simulink model "GFLI_L"  (R2024b)
settings: Solver=ode4  StartTime=0.0  StopTime=Tsim  FixedStep=Tsam  RelTol=1e-3
values from neighbouring files (symbols this model uses):
  Tsam = 5e-5    (= 5e-05)    [generate_ibr_impedance_datasets_param_casegrid_memorysafe.m]
  w_meas = 2*pi*fHz_meas(:)    [generate_ibr_impedance_datasets_param_casegrid_memorysafe.m]
undefined symbols (not defined in the file or in its folder): DiscIntNeverNeededParam, I2d, I2q, Kii, Kipll, Kpi, Kppll, Lf1, Rf1, Td, Vdc, Vg, w, w1
libraries: slctrl_fre x12, spsControlledVoltageSourceLib x6, spsabctodq0Lib x5, slctrl_signal x4, spsACVoltageSourceLib x3, spsSeriesRLCBranchLib x3, spsdq0toabcLib x2, spsThreePhaseVIMeasurementLib x2, spsPLL3phLib x1, spsGroundLib x1, sps_lib x1
(part 2 of 2)

== system GFLI_L/Data Logging for 'frestimate'1/Generate Info Signal/Superposition ==
  start/stop : Inport
  Info Bus : BusCreator  Inputs=1
  Info Snapshot : slctrl_fre/Frequency Response Estimator/Frequency Response Estimator/Variant Subsystem/PRBSNoEst/Info Snapshot  SystemSampleTime=-1  VariantActivationTime=update diagram  AllowFlexibleInterface=on  Latency=0  AutoFrameSizeCalculation=off
  conversion factor : Gain  Gain=ConvFactor
  frequencies : Constant  Value=FrequenciesSI  SampleTime=Ts
  Info : Outport
  wires:
  conversion factor/1 -> Info Snapshot/1
  Info Bus/1 -> Info/1  "Info"
  start/stop/1 -> Info Snapshot/Enable
  frequencies/1 -> conversion factor/1
  Info Snapshot/1 -> Info Bus/1  "frequencies"

== system GFLI_L/Data Logging for 'frestimate'1/Generate Ready Signal/PRBS ==
  Freq Index : Inport
  Perturbation : Inport  Port=2
  Constant : Constant  Value=0  SampleTime=Ts
  Relational Operator : RelationalOperator  Operator=~=  OutDataTypeStr=boolean  RndMeth=Simplest  InputSameDT=off
  Terminator : Terminator
  Ready : Outport
  wires:
  Relational Operator/1 -> Ready/1  "Ready"
  Constant/1 -> Relational Operator/2
  Perturbation/1 -> Relational Operator/1  "Perturbation"
  Freq Index/1 -> Terminator/1

== system GFLI_L/Data Logging for 'frestimate'1/Generate Ready Signal/Sinestream ==
  Freq Index : Inport
  Perturbation : Inport  Port=2
  ExtractReadySignal : Subsystem  mask(Extract Ready Signal){Ts=Ts, Frequencies=FrequenciesSS, NumOfSetPeriod=NumOfSetPeriod, NumOfEstPeriod=NumOfEstPeriod}
      mask prompts: Ts "Sample Time (Ts)"; Frequencies "Frequencies Vector"; NumOfSetPeriod "Number of Settling Periods"; NumOfEstPeriod "Number of Estimation Periods"
      mask help: Extract ready signal for the Sinestream Signal Generator block for offline frequency response estimation.
      mask init:
      | nw = length(Frequencies);
  Terminator : Terminator
  Ready : Outport
  wires:
  Freq Index/1 -> ExtractReadySignal/1(Frequency Index)
  Perturbation/1 -> Terminator/1
  ExtractReadySignal/1(Ready Signal) -> Ready/1  "Ready"

== system GFLI_L/Data Logging for 'frestimate'1/Generate Ready Signal/Superposition ==
  Freq Index : Inport
  Perturbation : Inport  Port=2
  Constant : Constant  Value=0  SampleTime=Ts
  Relational Operator : RelationalOperator  Operator=~=  OutDataTypeStr=boolean  RndMeth=Simplest  InputSameDT=off
  Terminator : Terminator
  Ready : Outport
  wires:
  Freq Index/1 -> Terminator/1
  Perturbation/1 -> Relational Operator/1  "Perturbation"
  Constant/1 -> Relational Operator/2
  Relational Operator/1 -> Ready/1  "Ready"

== system GFLI_L/Data Logging for 'frestimate'1/Subtract Nominal Values/Enabled Subsystem ==
  u : Inport
  y : Inport  Port=2
  start/stop : Inport  Port=3
  Enable : EnablePort
  ExtractNominalValues : Subsystem  mask(Remove Nominal Signal){Ts=Ts}
      mask prompts: Ts "Samplt Time (sec)"
      mask help: Remove nominal baseline signal from logged data.
  Sum : Sum  Inputs=|+-
  Sum1 : Sum  Inputs=-+|
  PlantInput : Outport
  PlantOutput : Outport  Port=2
  wires:
  Sum1/1 -> PlantOutput/1
  y/1 -> ExtractNominalValues/2(y), Sum1/2
  ExtractNominalValues/2(yNominal) -> Sum1/1
  u/1 -> ExtractNominalValues/1(u), Sum/1
  ExtractNominalValues/1(uNominal) -> Sum/2
  Sum/1 -> PlantInput/1
  start/stop/1 -> ExtractNominalValues/3(start/stop)

== system GFLI_L/Data Logging for 'frestimate'2/Generate Info Signal/PRBS ==
  start/stop : Inport
  Info Bus : BusCreator  Inputs=1
  Info Snapshot : slctrl_fre/Frequency Response Estimator/Frequency Response Estimator/Variant Subsystem/PRBSNoEst/Info Snapshot  SystemSampleTime=-1  VariantActivationTime=update diagram  AllowFlexibleInterface=on  Latency=0  AutoFrameSizeCalculation=off
  PRBSNumPeriods : Constant  Value=PRBSNumOfPeriod  SampleTime=Ts
  Info : Outport
  wires:
  PRBSNumPeriods/1 -> Info Snapshot/1
  Info Bus/1 -> Info/1  "Info"
  Info Snapshot/1 -> Info Bus/1  "PRBSNumPeriods"
  start/stop/1 -> Info Snapshot/Enable

== system GFLI_L/Data Logging for 'frestimate'2/Generate Info Signal/Sinestream ==
  start/stop : Inport
  Info Bus : BusCreator  Inputs=1
  Info Snapshot : slctrl_fre/Frequency Response Estimator/Frequency Response Estimator/Variant Subsystem/PRBSNoEst/Info Snapshot  SystemSampleTime=-1  VariantActivationTime=update diagram  AllowFlexibleInterface=on  Latency=0  AutoFrameSizeCalculation=off
  conversion factor : Gain  Gain=ConvFactor
  frequencies : Constant  Value=FrequenciesSS  SampleTime=Ts
  Info : Outport
  wires:
  conversion factor/1 -> Info Snapshot/1
  Info Snapshot/1 -> Info Bus/1  "frequencies"
  frequencies/1 -> conversion factor/1
  start/stop/1 -> Info Snapshot/Enable
  Info Bus/1 -> Info/1  "Info"

== system GFLI_L/Data Logging for 'frestimate'2/Generate Info Signal/Superposition ==
  start/stop : Inport
  Info Bus : BusCreator  Inputs=1
  Info Snapshot : slctrl_fre/Frequency Response Estimator/Frequency Response Estimator/Variant Subsystem/PRBSNoEst/Info Snapshot  SystemSampleTime=-1  VariantActivationTime=update diagram  AllowFlexibleInterface=on  Latency=0  AutoFrameSizeCalculation=off
  conversion factor : Gain  Gain=ConvFactor
  frequencies : Constant  Value=FrequenciesSI  SampleTime=Ts
  Info : Outport
  wires:
  conversion factor/1 -> Info Snapshot/1
  Info Bus/1 -> Info/1  "Info"
  start/stop/1 -> Info Snapshot/Enable
  frequencies/1 -> conversion factor/1
  Info Snapshot/1 -> Info Bus/1  "frequencies"

== system GFLI_L/Data Logging for 'frestimate'2/Generate Ready Signal/PRBS ==
  Freq Index : Inport
  Perturbation : Inport  Port=2
  Constant : Constant  Value=0  SampleTime=Ts
  Relational Operator : RelationalOperator  Operator=~=  OutDataTypeStr=boolean  RndMeth=Simplest  InputSameDT=off
  Terminator : Terminator
  Ready : Outport
  wires:
  Relational Operator/1 -> Ready/1  "Ready"
  Constant/1 -> Relational Operator/2
  Perturbation/1 -> Relational Operator/1  "Perturbation"
  Freq Index/1 -> Terminator/1

== system GFLI_L/Data Logging for 'frestimate'2/Generate Ready Signal/Sinestream ==
  Freq Index : Inport
  Perturbation : Inport  Port=2
  ExtractReadySignal : Subsystem  mask(Extract Ready Signal){Ts=Ts, Frequencies=FrequenciesSS, NumOfSetPeriod=NumOfSetPeriod, NumOfEstPeriod=NumOfEstPeriod}
      mask prompts: Ts "Sample Time (Ts)"; Frequencies "Frequencies Vector"; NumOfSetPeriod "Number of Settling Periods"; NumOfEstPeriod "Number of Estimation Periods"
      mask help: Extract ready signal for the Sinestream Signal Generator block for offline frequency response estimation.
      mask init:
      | nw = length(Frequencies);
  Terminator : Terminator
  Ready : Outport
  wires:
  Freq Index/1 -> ExtractReadySignal/1(Frequency Index)
  Perturbation/1 -> Terminator/1
  ExtractReadySignal/1(Ready Signal) -> Ready/1  "Ready"

== system GFLI_L/Data Logging for 'frestimate'2/Generate Ready Signal/Superposition ==
  Freq Index : Inport
  Perturbation : Inport  Port=2
  Constant : Constant  Value=0  SampleTime=Ts
  Relational Operator : RelationalOperator  Operator=~=  OutDataTypeStr=boolean  RndMeth=Simplest  InputSameDT=off
  Terminator : Terminator
  Ready : Outport
  wires:
  Freq Index/1 -> Terminator/1
  Perturbation/1 -> Relational Operator/1  "Perturbation"
  Constant/1 -> Relational Operator/2
  Relational Operator/1 -> Ready/1  "Ready"

== system GFLI_L/Data Logging for 'frestimate'2/Subtract Nominal Values/Enabled Subsystem ==
  u : Inport
  y : Inport  Port=2
  start/stop : Inport  Port=3
  Enable : EnablePort
  ExtractNominalValues : Subsystem  mask(Remove Nominal Signal){Ts=Ts}
      mask prompts: Ts "Samplt Time (sec)"
      mask help: Remove nominal baseline signal from logged data.
  Sum : Sum  Inputs=|+-
  Sum1 : Sum  Inputs=-+|
  PlantInput : Outport
  PlantOutput : Outport  Port=2
  wires:
  Sum1/1 -> PlantOutput/1
  y/1 -> ExtractNominalValues/2(y), Sum1/2
  ExtractNominalValues/2(yNominal) -> Sum1/1
  u/1 -> ExtractNominalValues/1(u), Sum/1
  ExtractNominalValues/1(uNominal) -> Sum/2
  Sum/1 -> PlantInput/1
  start/stop/1 -> ExtractNominalValues/3(start/stop)

== system GFLI_L/Data Logging for 'frestimate'3/Generate Info Signal/PRBS ==
  start/stop : Inport
  Info Bus : BusCreator  Inputs=1
  Info Snapshot : slctrl_fre/Frequency Response Estimator/Frequency Response Estimator/Variant Subsystem/PRBSNoEst/Info Snapshot  SystemSampleTime=-1  VariantActivationTime=update diagram  AllowFlexibleInterface=on  Latency=0  AutoFrameSizeCalculation=off
  PRBSNumPeriods : Constant  Value=PRBSNumOfPeriod  SampleTime=Ts
  Info : Outport
  wires:
  start/stop/1 -> Info Snapshot/Enable
  Info Snapshot/1 -> Info Bus/1  "PRBSNumPeriods"
  Info Bus/1 -> Info/1  "Info"
  PRBSNumPeriods/1 -> Info Snapshot/1

== system GFLI_L/Data Logging for 'frestimate'3/Generate Info Signal/Sinestream ==
  start/stop : Inport
  Info Bus : BusCreator  Inputs=1
  Info Snapshot : slctrl_fre/Frequency Response Estimator/Frequency Response Estimator/Variant Subsystem/PRBSNoEst/Info Snapshot  SystemSampleTime=-1  VariantActivationTime=update diagram  AllowFlexibleInterface=on  Latency=0  AutoFrameSizeCalculation=off
  conversion factor : Gain  Gain=ConvFactor
  frequencies : Constant  Value=FrequenciesSS  SampleTime=Ts
  Info : Outport
  wires:
  Info Bus/1 -> Info/1  "Info"
  start/stop/1 -> Info Snapshot/Enable
  frequencies/1 -> conversion factor/1
  Info Snapshot/1 -> Info Bus/1  "frequencies"
  conversion factor/1 -> Info Snapshot/1

== system GFLI_L/Data Logging for 'frestimate'3/Generate Info Signal/Superposition ==
  start/stop : Inport
  Info Bus : BusCreator  Inputs=1
  Info Snapshot : slctrl_fre/Frequency Response Estimator/Frequency Response Estimator/Variant Subsystem/PRBSNoEst/Info Snapshot  SystemSampleTime=-1  VariantActivationTime=update diagram  AllowFlexibleInterface=on  Latency=0  AutoFrameSizeCalculation=off
  conversion factor : Gain  Gain=ConvFactor
  frequencies : Constant  Value=FrequenciesSI  SampleTime=Ts
  Info : Outport
  wires:
  Info Snapshot/1 -> Info Bus/1  "frequencies"
  frequencies/1 -> conversion factor/1
  start/stop/1 -> Info Snapshot/Enable
  Info Bus/1 -> Info/1  "Info"
  conversion factor/1 -> Info Snapshot/1

== system GFLI_L/Data Logging for 'frestimate'3/Generate Ready Signal/PRBS ==
  Freq Index : Inport
  Perturbation : Inport  Port=2
  Constant : Constant  Value=0  SampleTime=Ts
  Relational Operator : RelationalOperator  Operator=~=  OutDataTypeStr=boolean  RndMeth=Simplest  InputSameDT=off
  Terminator : Terminator
  Ready : Outport
  wires:
  Freq Index/1 -> Terminator/1
  Perturbation/1 -> Relational Operator/1  "Perturbation"
  Constant/1 -> Relational Operator/2
  Relational Operator/1 -> Ready/1  "Ready"

== system GFLI_L/Data Logging for 'frestimate'3/Generate Ready Signal/Sinestream ==
  Freq Index : Inport
  Perturbation : Inport  Port=2
  ExtractReadySignal : Subsystem  mask(Extract Ready Signal){Ts=Ts, Frequencies=FrequenciesSS, NumOfSetPeriod=NumOfSetPeriod, NumOfEstPeriod=NumOfEstPeriod}
      mask prompts: Ts "Sample Time (Ts)"; Frequencies "Frequencies Vector"; NumOfSetPeriod "Number of Settling Periods"; NumOfEstPeriod "Number of Estimation Periods"
      mask help: Extract ready signal for the Sinestream Signal Generator block for offline frequency response estimation.
      mask init:
      | nw = length(Frequencies);
  Terminator : Terminator
  Ready : Outport
  wires:
  ExtractReadySignal/1(Ready Signal) -> Ready/1  "Ready"
  Perturbation/1 -> Terminator/1
  Freq Index/1 -> ExtractReadySignal/1(Frequency Index)

== system GFLI_L/Data Logging for 'frestimate'3/Generate Ready Signal/Superposition ==
  Freq Index : Inport
  Perturbation : Inport  Port=2
  Constant : Constant  Value=0  SampleTime=Ts
  Relational Operator : RelationalOperator  Operator=~=  OutDataTypeStr=boolean  RndMeth=Simplest  InputSameDT=off
  Terminator : Terminator
  Ready : Outport
  wires:
  Relational Operator/1 -> Ready/1  "Ready"
  Constant/1 -> Relational Operator/2
  Perturbation/1 -> Relational Operator/1  "Perturbation"
  Freq Index/1 -> Terminator/1

== system GFLI_L/Data Logging for 'frestimate'3/Subtract Nominal Values/Enabled Subsystem ==
  u : Inport
  y : Inport  Port=2
  start/stop : Inport  Port=3
  Enable : EnablePort
  ExtractNominalValues : Subsystem  mask(Remove Nominal Signal){Ts=Ts}
      mask prompts: Ts "Samplt Time (sec)"
      mask help: Remove nominal baseline signal from logged data.
  Sum : Sum  Inputs=|+-
  Sum1 : Sum  Inputs=-+|
  PlantInput : Outport
  PlantOutput : Outport  Port=2
  wires:
  start/stop/1 -> ExtractNominalValues/3(start/stop)
  Sum/1 -> PlantInput/1
  ExtractNominalValues/1(uNominal) -> Sum/2
  u/1 -> Sum/1, ExtractNominalValues/1(u)
  ExtractNominalValues/2(yNominal) -> Sum1/1
  y/1 -> Sum1/2, ExtractNominalValues/2(y)
  Sum1/1 -> PlantOutput/1

== system GFLI_L/Data Logging for 'frestimate'/Generate Ready Signal/Sinestream/ExtractReadySignal ==
  Frequency Index : Inport
  Est Period : Constant  Value=NumOfEstPeriod  OutDataTypeStr=double
  MATLAB Function : MATLAB Function  TreatAsAtomicUnit=on
  Numest Scalar Expansion : Gain  Gain=ones(nw,1)
  Numset Scalar Expansion : Gain  Gain=ones(nw,1)
  Set Period : Constant  Value=NumOfSetPeriod  OutDataTypeStr=double
  Triggered Subsystem : Subsystem  TreatAsAtomicUnit=on
  sample time : Constant  Value=Ts  OutDataTypeStr=double
  w constant : Constant  Value=FrequenciesSS  OutDataTypeStr=double
  Ready Signal : Outport
  wires:
  sample time/1 -> MATLAB Function/2(Ts)
  Numest Scalar Expansion/1 -> MATLAB Function/3(NumOfEstPeriod)
  w constant/1 -> MATLAB Function/1(Frequencies)
  MATLAB Function/1(Tf) -> Triggered Subsystem/2(Tf)
  Est Period/1 -> Numest Scalar Expansion/1
  Numset Scalar Expansion/1 -> MATLAB Function/4(NumOfSetPeriod)
  Frequency Index/1 -> Triggered Subsystem/1(index), Triggered Subsystem/Enable
  Triggered Subsystem/1(Ready) -> Ready Signal/1
  Set Period/1 -> Numset Scalar Expansion/1
  MATLAB Function/2(tstart) -> Triggered Subsystem/3(tstart)
  MATLAB Function/3(tsettling) -> Triggered Subsystem/4(tsettling)

== system GFLI_L/Data Logging for 'frestimate'/Subtract Nominal Values/Enabled Subsystem/ExtractNominalValues ==
  u : Inport
  y : Inport  Port=2
  start/stop : Inport  Port=3
  DisplayU0 : Display
  DisplayY0 : Display
  Enabled Delay U : Delay  DelayLength=1  InitialConditionSource=Input port  ExternalReset=Rising  SampleTime=Ts
      settings: InputPortMap=u0,r5,p4
  Enabled Delay Y : Delay  DelayLength=1  InitialConditionSource=Input port  ExternalReset=Rising  SampleTime=Ts
      settings: InputPortMap=u0,r5,p4
  uNominal : Outport  OutDataTypeStr=double  VectorParamsAs1DForOutWhenUnconnected=off
  yNominal : Outport  Port=2  OutDataTypeStr=double  VectorParamsAs1DForOutWhenUnconnected=off
  wires:
  Enabled Delay U/1 -> uNominal/1, DisplayU0/1, Enabled Delay U/1  "u"
  Enabled Delay Y/1 -> yNominal/1, Enabled Delay Y/1, DisplayY0/1  "y"
  start/stop/1 -> Enabled Delay Y/2, Enabled Delay U/2
  u/1 -> Enabled Delay U/3
  y/1 -> Enabled Delay Y/3

== system GFLI_L/Data Logging for 'frestimate'1/Generate Ready Signal/Sinestream/ExtractReadySignal ==
  Frequency Index : Inport
  Est Period : Constant  Value=NumOfEstPeriod  OutDataTypeStr=double
  MATLAB Function : MATLAB Function  TreatAsAtomicUnit=on
  Numest Scalar Expansion : Gain  Gain=ones(nw,1)
  Numset Scalar Expansion : Gain  Gain=ones(nw,1)
  Set Period : Constant  Value=NumOfSetPeriod  OutDataTypeStr=double
  Triggered Subsystem : Subsystem  TreatAsAtomicUnit=on
  sample time : Constant  Value=Ts  OutDataTypeStr=double
  w constant : Constant  Value=FrequenciesSS  OutDataTypeStr=double
  Ready Signal : Outport
  wires:
  MATLAB Function/3(tsettling) -> Triggered Subsystem/4(tsettling)
  MATLAB Function/2(tstart) -> Triggered Subsystem/3(tstart)
  Set Period/1 -> Numset Scalar Expansion/1
  Triggered Subsystem/1(Ready) -> Ready Signal/1
  Frequency Index/1 -> Triggered Subsystem/Enable, Triggered Subsystem/1(index)
  Numset Scalar Expansion/1 -> MATLAB Function/4(NumOfSetPeriod)
  Est Period/1 -> Numest Scalar Expansion/1
  MATLAB Function/1(Tf) -> Triggered Subsystem/2(Tf)
  w constant/1 -> MATLAB Function/1(Frequencies)
  Numest Scalar Expansion/1 -> MATLAB Function/3(NumOfEstPeriod)
  sample time/1 -> MATLAB Function/2(Ts)

== system GFLI_L/Data Logging for 'frestimate'1/Subtract Nominal Values/Enabled Subsystem/ExtractNominalValues ==
  u : Inport
  y : Inport  Port=2
  start/stop : Inport  Port=3
  DisplayU0 : Display
  DisplayY0 : Display
  Enabled Delay U : Delay  DelayLength=1  InitialConditionSource=Input port  ExternalReset=Rising  SampleTime=Ts
      settings: InputPortMap=u0,r5,p4
  Enabled Delay Y : Delay  DelayLength=1  InitialConditionSource=Input port  ExternalReset=Rising  SampleTime=Ts
      settings: InputPortMap=u0,r5,p4
  uNominal : Outport  OutDataTypeStr=double  VectorParamsAs1DForOutWhenUnconnected=off
  yNominal : Outport  Port=2  OutDataTypeStr=double  VectorParamsAs1DForOutWhenUnconnected=off
  wires:
  y/1 -> Enabled Delay Y/3
  u/1 -> Enabled Delay U/3
  start/stop/1 -> Enabled Delay U/2, Enabled Delay Y/2
  Enabled Delay Y/1 -> DisplayY0/1, Enabled Delay Y/1, yNominal/1  "y"
  Enabled Delay U/1 -> Enabled Delay U/1, DisplayU0/1, uNominal/1  "u"

== system GFLI_L/Data Logging for 'frestimate'2/Generate Ready Signal/Sinestream/ExtractReadySignal ==
  Frequency Index : Inport
  Est Period : Constant  Value=NumOfEstPeriod  OutDataTypeStr=double
  MATLAB Function : MATLAB Function  TreatAsAtomicUnit=on
  Numest Scalar Expansion : Gain  Gain=ones(nw,1)
  Numset Scalar Expansion : Gain  Gain=ones(nw,1)
  Set Period : Constant  Value=NumOfSetPeriod  OutDataTypeStr=double
  Triggered Subsystem : Subsystem  TreatAsAtomicUnit=on
  sample time : Constant  Value=Ts  OutDataTypeStr=double
  w constant : Constant  Value=FrequenciesSS  OutDataTypeStr=double
  Ready Signal : Outport
  wires:
  MATLAB Function/3(tsettling) -> Triggered Subsystem/4(tsettling)
  MATLAB Function/2(tstart) -> Triggered Subsystem/3(tstart)
  Set Period/1 -> Numset Scalar Expansion/1
  Triggered Subsystem/1(Ready) -> Ready Signal/1
  Frequency Index/1 -> Triggered Subsystem/Enable, Triggered Subsystem/1(index)
  Numset Scalar Expansion/1 -> MATLAB Function/4(NumOfSetPeriod)
  Est Period/1 -> Numest Scalar Expansion/1
  MATLAB Function/1(Tf) -> Triggered Subsystem/2(Tf)
  w constant/1 -> MATLAB Function/1(Frequencies)
  Numest Scalar Expansion/1 -> MATLAB Function/3(NumOfEstPeriod)
  sample time/1 -> MATLAB Function/2(Ts)

== system GFLI_L/Data Logging for 'frestimate'2/Subtract Nominal Values/Enabled Subsystem/ExtractNominalValues ==
  u : Inport
  y : Inport  Port=2
  start/stop : Inport  Port=3
  DisplayU0 : Display
  DisplayY0 : Display
  Enabled Delay U : Delay  DelayLength=1  InitialConditionSource=Input port  ExternalReset=Rising  SampleTime=Ts
      settings: InputPortMap=u0,r5,p4
  Enabled Delay Y : Delay  DelayLength=1  InitialConditionSource=Input port  ExternalReset=Rising  SampleTime=Ts
      settings: InputPortMap=u0,r5,p4
  uNominal : Outport  OutDataTypeStr=double  VectorParamsAs1DForOutWhenUnconnected=off
  yNominal : Outport  Port=2  OutDataTypeStr=double  VectorParamsAs1DForOutWhenUnconnected=off
  wires:
  y/1 -> Enabled Delay Y/3
  u/1 -> Enabled Delay U/3
  start/stop/1 -> Enabled Delay U/2, Enabled Delay Y/2
  Enabled Delay Y/1 -> DisplayY0/1, Enabled Delay Y/1, yNominal/1  "y"
  Enabled Delay U/1 -> Enabled Delay U/1, DisplayU0/1, uNominal/1  "u"

== system GFLI_L/Data Logging for 'frestimate'3/Generate Ready Signal/Sinestream/ExtractReadySignal ==
  Frequency Index : Inport
  Est Period : Constant  Value=NumOfEstPeriod  OutDataTypeStr=double
  MATLAB Function : MATLAB Function  TreatAsAtomicUnit=on
  Numest Scalar Expansion : Gain  Gain=ones(nw,1)
  Numset Scalar Expansion : Gain  Gain=ones(nw,1)
  Set Period : Constant  Value=NumOfSetPeriod  OutDataTypeStr=double
  Triggered Subsystem : Subsystem  TreatAsAtomicUnit=on
  sample time : Constant  Value=Ts  OutDataTypeStr=double
  w constant : Constant  Value=FrequenciesSS  OutDataTypeStr=double
  Ready Signal : Outport
  wires:
  sample time/1 -> MATLAB Function/2(Ts)
  Numest Scalar Expansion/1 -> MATLAB Function/3(NumOfEstPeriod)
  w constant/1 -> MATLAB Function/1(Frequencies)
  MATLAB Function/1(Tf) -> Triggered Subsystem/2(Tf)
  Est Period/1 -> Numest Scalar Expansion/1
  Numset Scalar Expansion/1 -> MATLAB Function/4(NumOfSetPeriod)
  Frequency Index/1 -> Triggered Subsystem/1(index), Triggered Subsystem/Enable
  Triggered Subsystem/1(Ready) -> Ready Signal/1
  Set Period/1 -> Numset Scalar Expansion/1
  MATLAB Function/2(tstart) -> Triggered Subsystem/3(tstart)
  MATLAB Function/3(tsettling) -> Triggered Subsystem/4(tsettling)

== system GFLI_L/Data Logging for 'frestimate'3/Subtract Nominal Values/Enabled Subsystem/ExtractNominalValues ==
  u : Inport
  y : Inport  Port=2
  start/stop : Inport  Port=3
  DisplayU0 : Display
  DisplayY0 : Display
  Enabled Delay U : Delay  DelayLength=1  InitialConditionSource=Input port  ExternalReset=Rising  SampleTime=Ts
      settings: InputPortMap=u0,r5,p4
  Enabled Delay Y : Delay  DelayLength=1  InitialConditionSource=Input port  ExternalReset=Rising  SampleTime=Ts
      settings: InputPortMap=u0,r5,p4
  uNominal : Outport  OutDataTypeStr=double  VectorParamsAs1DForOutWhenUnconnected=off
  yNominal : Outport  Port=2  OutDataTypeStr=double  VectorParamsAs1DForOutWhenUnconnected=off
  wires:
  Enabled Delay U/1 -> uNominal/1, DisplayU0/1, Enabled Delay U/1  "u"
  Enabled Delay Y/1 -> yNominal/1, Enabled Delay Y/1, DisplayY0/1  "y"
  start/stop/1 -> Enabled Delay Y/2, Enabled Delay U/2
  u/1 -> Enabled Delay U/3
  y/1 -> Enabled Delay Y/3

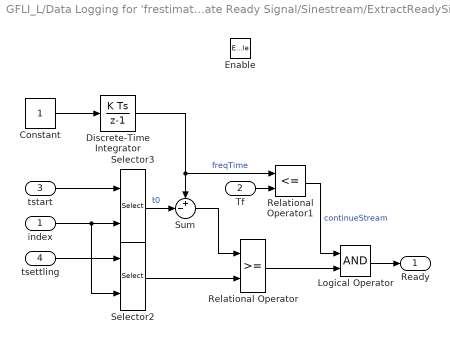
== system GFLI_L/Data Logging for 'frestimate'/Generate Ready Signal/Sinestream/ExtractReadySignal/Triggered Subsystem ==
  index : Inport
  Tf : Inport  Port=2
  tstart : Inport  Port=3
  tsettling : Inport  Port=4
  Enable : EnablePort
  Constant : Constant  OutDataTypeStr=double
  Discrete-Time Integrator : DiscreteIntegrator  SampleTime=Ts  ICPrevOutput=DiscIntNeverNeededParam  ICPrevScaledInput=DiscIntNeverNeededParam
  Logical Operator : Logic  AllPortsSameDT=off  OutDataTypeStr=boolean
  Relational Operator : RelationalOperator  OutDataTypeStr=boolean  RndMeth=Simplest  InputSameDT=off
  Relational Operator1 : RelationalOperator  Operator=<=  OutDataTypeStr=boolean  RndMeth=Simplest  InputSameDT=off
  Selector2 : Selector  InputPortWidth=nw  IndexOptions=Index vector (port)  Indices=[1 3]  OutputSizes=1
  Selector3 : Selector  InputPortWidth=nw  IndexOptions=Index vector (port)  Indices=[1 3]  OutputSizes=1
  Sum : Sum  Inputs=+-|
  Ready : Outport
  wires:
  Constant/1 -> Discrete-Time Integrator/1
  Sum/1 -> Relational Operator/1
  tstart/1 -> Selector3/1
  tsettling/1 -> Selector2/1
  Selector2/1 -> Relational Operator/2
  Selector3/1 -> Sum/2  "t0"
  Discrete-Time Integrator/1 -> Sum/1, Relational Operator1/1  "freqTime"
  index/1 -> Selector2/2, Selector3/2
  Relational Operator/1 -> Logical Operator/2
  Tf/1 -> Relational Operator1/2
  Relational Operator1/1 -> Logical Operator/1  "continueStream"
  Logical Operator/1 -> Ready/1

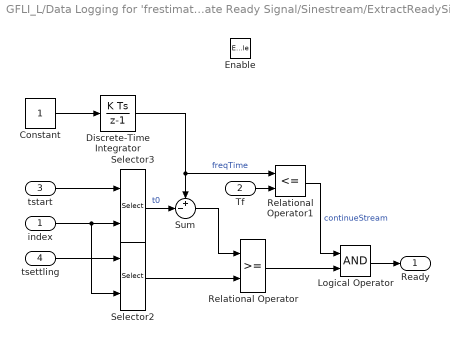
== system GFLI_L/Data Logging for 'frestimate'1/Generate Ready Signal/Sinestream/ExtractReadySignal/Triggered Subsystem ==
  index : Inport
  Tf : Inport  Port=2
  tstart : Inport  Port=3
  tsettling : Inport  Port=4
  Enable : EnablePort
  Constant : Constant  OutDataTypeStr=double
  Discrete-Time Integrator : DiscreteIntegrator  SampleTime=Ts  ICPrevOutput=DiscIntNeverNeededParam  ICPrevScaledInput=DiscIntNeverNeededParam
  Logical Operator : Logic  AllPortsSameDT=off  OutDataTypeStr=boolean
  Relational Operator : RelationalOperator  OutDataTypeStr=boolean  RndMeth=Simplest  InputSameDT=off
  Relational Operator1 : RelationalOperator  Operator=<=  OutDataTypeStr=boolean  RndMeth=Simplest  InputSameDT=off
  Selector2 : Selector  InputPortWidth=nw  IndexOptions=Index vector (port)  Indices=[1 3]  OutputSizes=1
  Selector3 : Selector  InputPortWidth=nw  IndexOptions=Index vector (port)  Indices=[1 3]  OutputSizes=1
  Sum : Sum  Inputs=+-|
  Ready : Outport
  wires:
  Logical Operator/1 -> Ready/1
  Relational Operator1/1 -> Logical Operator/1  "continueStream"
  Tf/1 -> Relational Operator1/2
  Relational Operator/1 -> Logical Operator/2
  index/1 -> Selector3/2, Selector2/2
  Discrete-Time Integrator/1 -> Relational Operator1/1, Sum/1  "freqTime"
  Selector3/1 -> Sum/2  "t0"
  Selector2/1 -> Relational Operator/2
  tsettling/1 -> Selector2/1
  tstart/1 -> Selector3/1
  Sum/1 -> Relational Operator/1
  Constant/1 -> Discrete-Time Integrator/1

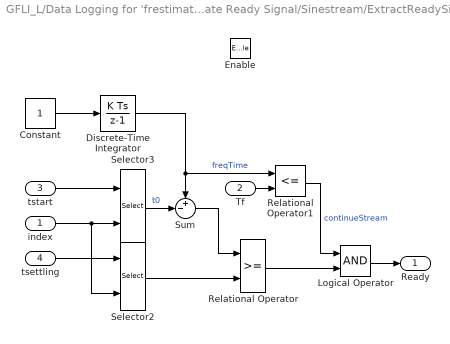
== system GFLI_L/Data Logging for 'frestimate'2/Generate Ready Signal/Sinestream/ExtractReadySignal/Triggered Subsystem ==
  index : Inport
  Tf : Inport  Port=2
  tstart : Inport  Port=3
  tsettling : Inport  Port=4
  Enable : EnablePort
  Constant : Constant  OutDataTypeStr=double
  Discrete-Time Integrator : DiscreteIntegrator  SampleTime=Ts  ICPrevOutput=DiscIntNeverNeededParam  ICPrevScaledInput=DiscIntNeverNeededParam
  Logical Operator : Logic  AllPortsSameDT=off  OutDataTypeStr=boolean
  Relational Operator : RelationalOperator  OutDataTypeStr=boolean  RndMeth=Simplest  InputSameDT=off
  Relational Operator1 : RelationalOperator  Operator=<=  OutDataTypeStr=boolean  RndMeth=Simplest  InputSameDT=off
  Selector2 : Selector  InputPortWidth=nw  IndexOptions=Index vector (port)  Indices=[1 3]  OutputSizes=1
  Selector3 : Selector  InputPortWidth=nw  IndexOptions=Index vector (port)  Indices=[1 3]  OutputSizes=1
  Sum : Sum  Inputs=+-|
  Ready : Outport
  wires:
  Logical Operator/1 -> Ready/1
  Relational Operator1/1 -> Logical Operator/1  "continueStream"
  Tf/1 -> Relational Operator1/2
  Relational Operator/1 -> Logical Operator/2
  index/1 -> Selector3/2, Selector2/2
  Discrete-Time Integrator/1 -> Relational Operator1/1, Sum/1  "freqTime"
  Selector3/1 -> Sum/2  "t0"
  Selector2/1 -> Relational Operator/2
  tsettling/1 -> Selector2/1
  tstart/1 -> Selector3/1
  Sum/1 -> Relational Operator/1
  Constant/1 -> Discrete-Time Integrator/1

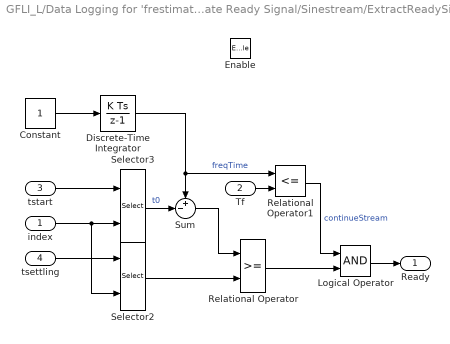
== system GFLI_L/Data Logging for 'frestimate'3/Generate Ready Signal/Sinestream/ExtractReadySignal/Triggered Subsystem ==
  index : Inport
  Tf : Inport  Port=2
  tstart : Inport  Port=3
  tsettling : Inport  Port=4
  Enable : EnablePort
  Constant : Constant  OutDataTypeStr=double
  Discrete-Time Integrator : DiscreteIntegrator  SampleTime=Ts  ICPrevOutput=DiscIntNeverNeededParam  ICPrevScaledInput=DiscIntNeverNeededParam
  Logical Operator : Logic  AllPortsSameDT=off  OutDataTypeStr=boolean
  Relational Operator : RelationalOperator  OutDataTypeStr=boolean  RndMeth=Simplest  InputSameDT=off
  Relational Operator1 : RelationalOperator  Operator=<=  OutDataTypeStr=boolean  RndMeth=Simplest  InputSameDT=off
  Selector2 : Selector  InputPortWidth=nw  IndexOptions=Index vector (port)  Indices=[1 3]  OutputSizes=1
  Selector3 : Selector  InputPortWidth=nw  IndexOptions=Index vector (port)  Indices=[1 3]  OutputSizes=1
  Sum : Sum  Inputs=+-|
  Ready : Outport
  wires:
  Constant/1 -> Discrete-Time Integrator/1
  Sum/1 -> Relational Operator/1
  tstart/1 -> Selector3/1
  tsettling/1 -> Selector2/1
  Selector2/1 -> Relational Operator/2
  Selector3/1 -> Sum/2  "t0"
  Discrete-Time Integrator/1 -> Sum/1, Relational Operator1/1  "freqTime"
  index/1 -> Selector2/2, Selector3/2
  Relational Operator/1 -> Logical Operator/2
  Tf/1 -> Relational Operator1/2
  Relational Operator1/1 -> Logical Operator/1  "continueStream"
  Logical Operator/1 -> Ready/1

== matlab function GFLI_L/Data Logging for 'frestimate'/Generate Ready Signal/Sinestream/ExtractReadySignal/MATLAB Function ==
  data: Frequencies input; Tf output; Ts input; NumOfEstPeriod input; NumOfSetPeriod input; tstart output; tsettling output
function [Tf, tstart, tsettling] = extractReadySignal(Frequencies,Ts,NumOfEstPeriod,NumOfSetPeriod)
% obtain the number of periods requested for each frequency
NumPeriods = NumOfEstPeriod + NumOfSetPeriod;
% obtain period time for each frequency
T = 2*pi./Frequencies;
% define experiment length for each frequency (add two samples for CA)
Length = NumPeriods.*T+2*Ts;
% calculate start time stamp for each frequency
CUMSUM = cumsum(Length);
tstart = [0;CUMSUM(1:end-1)];
% calculate the settling duration for each frequency (cannot be zero)
tsettling = [NumOfSetPeriod.*T];
% obtain the stop time for the experiment
Tf = CUMSUM(end);

== matlab function GFLI_L/Data Logging for 'frestimate'1/Generate Ready Signal/Sinestream/ExtractReadySignal/MATLAB Function ==
  data: Frequencies input; Tf output; Ts input; NumOfEstPeriod input; NumOfSetPeriod input; tstart output; tsettling output
function [Tf, tstart, tsettling] = extractReadySignal(Frequencies,Ts,NumOfEstPeriod,NumOfSetPeriod)
% obtain the number of periods requested for each frequency
NumPeriods = NumOfEstPeriod + NumOfSetPeriod;
% obtain period time for each frequency
T = 2*pi./Frequencies;
% define experiment length for each frequency (add two samples for CA)
Length = NumPeriods.*T+2*Ts;
% calculate start time stamp for each frequency
CUMSUM = cumsum(Length);
tstart = [0;CUMSUM(1:end-1)];
% calculate the settling duration for each frequency (cannot be zero)
tsettling = [NumOfSetPeriod.*T];
% obtain the stop time for the experiment
Tf = CUMSUM(end);

== matlab function GFLI_L/Data Logging for 'frestimate'2/Generate Ready Signal/Sinestream/ExtractReadySignal/MATLAB Function ==
  data: Frequencies input; Tf output; Ts input; NumOfEstPeriod input; NumOfSetPeriod input; tstart output; tsettling output
function [Tf, tstart, tsettling] = extractReadySignal(Frequencies,Ts,NumOfEstPeriod,NumOfSetPeriod)
% obtain the number of periods requested for each frequency
NumPeriods = NumOfEstPeriod + NumOfSetPeriod;
% obtain period time for each frequency
T = 2*pi./Frequencies;
% define experiment length for each frequency (add two samples for CA)
Length = NumPeriods.*T+2*Ts;
% calculate start time stamp for each frequency
CUMSUM = cumsum(Length);
tstart = [0;CUMSUM(1:end-1)];
% calculate the settling duration for each frequency (cannot be zero)
tsettling = [NumOfSetPeriod.*T];
% obtain the stop time for the experiment
Tf = CUMSUM(end);

== matlab function GFLI_L/Data Logging for 'frestimate'3/Generate Ready Signal/Sinestream/ExtractReadySignal/MATLAB Function ==
  data: Frequencies input; Tf output; Ts input; NumOfEstPeriod input; NumOfSetPeriod input; tstart output; tsettling output
function [Tf, tstart, tsettling] = extractReadySignal(Frequencies,Ts,NumOfEstPeriod,NumOfSetPeriod)
% obtain the number of periods requested for each frequency
NumPeriods = NumOfEstPeriod + NumOfSetPeriod;
% obtain period time for each frequency
T = 2*pi./Frequencies;
% define experiment length for each frequency (add two samples for CA)
Length = NumPeriods.*T+2*Ts;
% calculate start time stamp for each frequency
CUMSUM = cumsum(Length);
tstart = [0;CUMSUM(1:end-1)];
% calculate the settling duration for each frequency (cannot be zero)
tsettling = [NumOfSetPeriod.*T];
% obtain the stop time for the experiment
Tf = CUMSUM(end);
